simulink model "nonlin_feedback_simInput"  (R2023a)
settings: Solver=ode1  StartTime=0  StopTime=400  FixedStep=0.002  RelTol=1e-3
values from neighbouring files (symbols this model uses):
  B1 = [-kQ, -kQ, kQ, kQ ... (first row only)    [simulate_hover.m]
  B2 = [0, 0, 0 ... (first row only)    [simulate_hover.m]
  cycleGain = 0.2    [simulate_hover.m]    (also in temp.m = 1)
  I_xx = 0.0522    [simulate_hover.m]
  I_yy = 0.0522    [simulate_hover.m]
  I_zz = 0.1104    [simulate_hover.m]
  K = lqi(sys, Q, R)    [simulate_hover.m]
  k_T = 0.1188    [simulate_hover.m]
  kd = 0.5    [simulate_hover.m]
  kfr_p = 0.4*u2line/x5line    (= 0.285774113641)    [simulate_hover.m]
  kfr_r = 0.4*u1line/x4line    (= 0.285774113641)    [simulate_hover.m]
  kfr_y = 0.4*u3line/x6line    (= 0.0880063173321)    [simulate_hover.m]
  l_a = 0.1968    [simulate_hover.m]
  r = flexSize(no)    [phaseComp.m]    (also in simulate_hover.m = 0.5)
  sigma = 0    [simulate_hover.m]
  skew = 2    [simulate_hover.m]
  V_bias = 12    [setup_lab_hover.m]    (also in simulate_hover.m)
  velMax = 100*60*pi/180    (= 104.71975512)    [simulate_hover.m]
  VMAX_AMP = 24    [setup_lab_hover.m]    (also in simulate_hover.m)
  wcf = 2 * pi * 20    (= 125.663706144)    [setup_lab_hover.m]    (also in simulate_hover.m)
  zetaf = 0.6    [setup_lab_hover.m]    (also in simulate_hover.m)
undefined symbols (not defined in the file or in its folder): DG
libraries: simulink_extras x4, dspsrcs4 x1
settings Model: Creator=kille  LastModifiedBy=Jacob

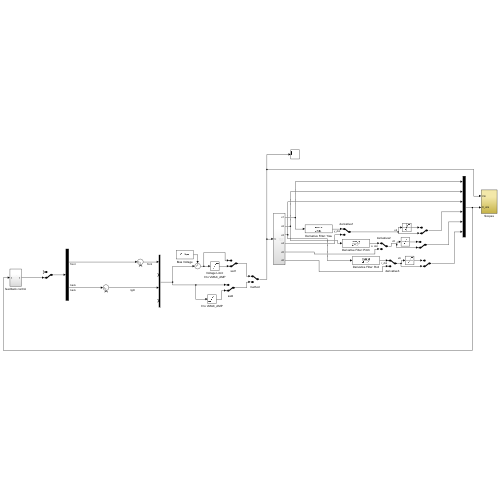
[thumbnail: Simulink's stored preview of the top-level diagram]
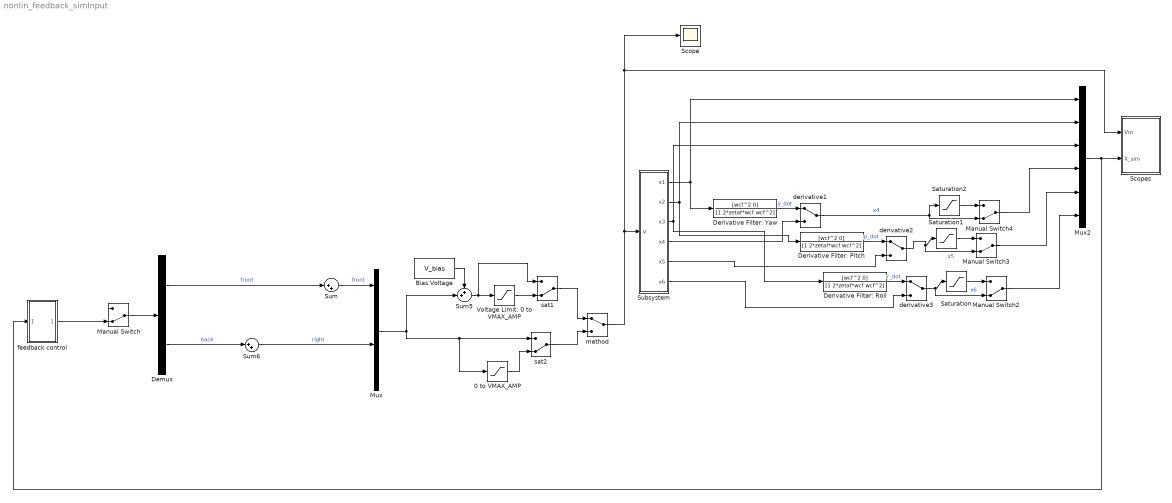
== system nonlin_feedback_simInput ==
  0 to VMAX_AMP : Saturate  UpperLimit=VMAX_AMP  LowerLimit=0
  Bias Voltage : Constant  Value=V_bias
  Demux : Demux  Outputs=2
  Derivative Filter: Pitch : TransferFcn  Numerator=[wcf^2 0]  Denominator=[1 2*zetaf*wcf wcf^2]
  Derivative Filter: Roll : TransferFcn  Numerator=[wcf^2 0]  Denominator=[1 2*zetaf*wcf wcf^2]
  Derivative Filter: Yaw : TransferFcn  Numerator=[wcf^2 0]  Denominator=[1 2*zetaf*wcf wcf^2]
  Manual Switch{,2..4} (4 alike) : ManualSwitch  CurrentSetting=0
  Mux : Mux
  Mux2 : Mux  Inputs=6
  Saturation : Saturate  UpperLimit=velMax  LowerLimit=-velMax
  Saturation1 : Saturate  UpperLimit=velMax  LowerLimit=-velMax
  Saturation2 : Saturate  UpperLimit=velMax  LowerLimit=-velMax
  Scope : Scope
  Scopes : Subsystem
  Subsystem : Subsystem
  Sum : Sum  Inputs=|++
  Sum5 : Sum  Inputs=++|
  Sum6 : Sum  Inputs=|++
  Voltage Limit: 0 to VMAX_AMP : Saturate  UpperLimit=VMAX_AMP  LowerLimit=0
  derivative1 : ManualSwitch
  derivative2 : ManualSwitch
  derivative3 : ManualSwitch
  feedback control : Subsystem
  method : ManualSwitch  Tag=swt
  sat1 : ManualSwitch  CurrentSetting=0
  sat2 : ManualSwitch  CurrentSetting=0
  wires:
  method/1 -> Scope/1, Scopes/1(Vm), Subsystem/1(V)
  sat2/1 -> method/2
  Mux/1 -> 0 to VMAX_AMP/1, sat2/1, Sum5/2
  Voltage Limit: 0 to VMAX_AMP/1 -> sat1/2
  Bias Voltage/1 -> Sum5/1
  Sum5/1 -> sat1/1, Voltage Limit: 0 to VMAX_AMP/1
  0 to VMAX_AMP/1 -> sat2/2
  sat1/1 -> method/1
  Sum/1 -> Mux/1  "front"
  Demux/1 -> Sum/1  "front"
  Sum6/1 -> Mux/3  "right"
  Derivative Filter: Yaw/1 -> derivative1/1  "y_dot"
  Derivative Filter: Pitch/1 -> derivative2/1  "p_dot"
  Derivative Filter: Roll/1 -> derivative3/1  "r_dot"
  Subsystem/1(x1) -> Mux2/1, Derivative Filter: Yaw/1
  Subsystem/4(x4) -> derivative1/2
  Subsystem/2(x2) -> Derivative Filter: Pitch/1, Mux2/2
  Subsystem/5(x5) -> derivative2/2
  Subsystem/6(x6) -> derivative3/2
  Subsystem/3(x3) -> Mux2/3, Derivative Filter: Roll/1
  Manual Switch4/1 -> Mux2/4
  Manual Switch2/1 -> Mux2/6
  Manual Switch3/1 -> Mux2/5
  Saturation/1 -> Manual Switch2/1
  derivative3/1 -> Manual Switch2/2, Saturation/1  "x6"
  Saturation1/1 -> Manual Switch3/1
  derivative2/1 -> Manual Switch3/2, Saturation1/1  "x5"
  Saturation2/1 -> Manual Switch4/1
  derivative1/1 -> Saturation2/1, Manual Switch4/2  "x4"
  Mux2/1 -> feedback control/1(In1), Scopes/2(X_sim)
  Demux/2 -> Sum6/1  "back"
  Manual Switch/1 -> Demux/1
  feedback control/1(Out1) -> Manual Switch/2

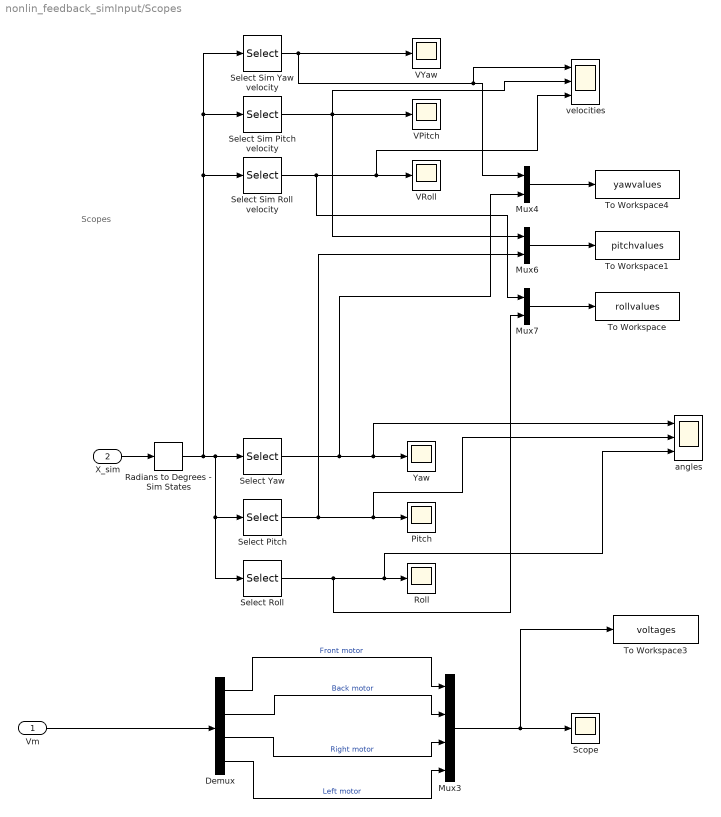
== system nonlin_feedback_simInput/Scopes ==
  note: Scopes
  Vm : Inport
  X_sim : Inport  Port=2
  Demux : Demux
  Mux3 : Mux
  Mux4 : Mux  Inputs=2
  Mux6 : Mux  Inputs=2
  Mux7 : Mux  Inputs=2
  Pitch : Scope
  Radians to Degrees - Sim States : simulink_extras/Transformations/Radians to Degrees
  Roll : Scope
  Scope : Scope
  Select Pitch : Selector  InputPortWidth=6  IndexOptions=Index vector (dialog)  Indices=2  OutputSizes=1
  Select Roll : Selector  InputPortWidth=6  IndexOptions=Index vector (dialog)  Indices=3  OutputSizes=1
  Select Sim Pitch velocity : Selector  InputPortWidth=6  IndexOptions=Index vector (dialog)  Indices=5  OutputSizes=1
  Select Sim Roll velocity : Selector  InputPortWidth=6  IndexOptions=Index vector (dialog)  Indices=6  OutputSizes=1
  Select Sim Yaw velocity : Selector  InputPortWidth=6  IndexOptions=Index vector (dialog)  Indices=4  OutputSizes=1
  Select Yaw : Selector  InputPortWidth=6  IndexOptions=Index vector (dialog)  Indices=1  OutputSizes=1
  To Workspace : ToWorkspace  VariableName=rollvalues  SampleTime=-1
  To Workspace1 : ToWorkspace  VariableName=pitchvalues  SampleTime=-1
  To Workspace3 : ToWorkspace  VariableName=voltages  SampleTime=-1
  To Workspace4 : ToWorkspace  VariableName=yawvalues  SampleTime=-1
  VPitch : Scope
  VRoll : Scope
  VYaw : Scope
  Yaw : Scope
  angles : Scope  NumInputPorts=3
  velocities : Scope  NumInputPorts=3
  wires:
  Select Roll/1 -> angles/3, Roll/1, Mux7/2
  Radians to Degrees - Sim States/1 -> Select Sim Roll velocity/1, Select Sim Pitch velocity/1, Select Sim Yaw velocity/1, Select Roll/1, Select Pitch/1, Select Yaw/1
  Select Pitch/1 -> angles/2, Pitch/1, Mux6/2
  X_sim/1 -> Radians to Degrees - Sim States/1
  Demux/1 -> Mux3/1  "Front motor"
  Demux/2 -> Mux3/2  "Back motor"
  Demux/3 -> Mux3/3  "Right motor"
  Demux/4 -> Mux3/4  "Left motor"
  Vm/1 -> Demux/1
  Select Sim Yaw velocity/1 -> VYaw/1, velocities/1, Mux4/1
  Select Sim Roll velocity/1 -> velocities/3, VRoll/1, Mux7/1
  Select Sim Pitch velocity/1 -> Mux6/1, velocities/2, VPitch/1
  Mux4/1 -> To Workspace4/1
  Mux6/1 -> To Workspace1/1
  Mux7/1 -> To Workspace/1
  Mux3/1 -> To Workspace3/1, Scope/1
  Select Yaw/1 -> angles/1, Yaw/1, Mux4/2

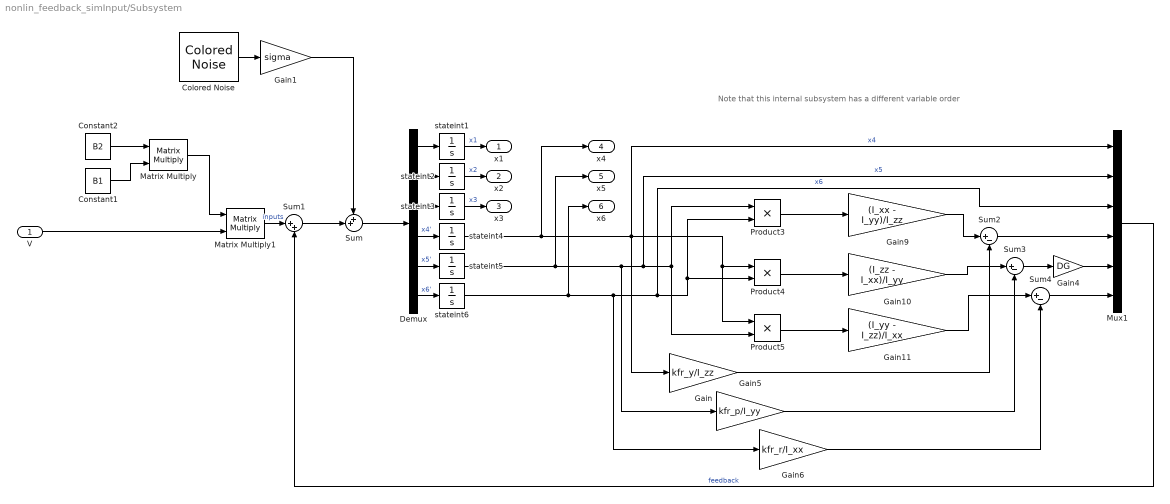
== system nonlin_feedback_simInput/Subsystem ==
  note: Note that this internal subsystem has a different variable order
  V : Inport
  Colored Noise : dspsrcs4/Colored Noise  Color=white  InverseFrequencyPower=1  BoundedOutput=off  NumChannels=6  OutputDataType=double  SamplesPerFrame=1  SampleTime=1  RandomStream=mt19937ar with seed  Seed=67  SimulateUsing=Interpreted execution
  Constant1 : Constant  Value=B1
  Constant2 : Constant  Value=B2
  Demux : Demux  Outputs=6
  Gain : Gain  Gain=kfr_y/I_zz
  Gain1 : Gain  Gain=sigma
  Gain10 : Gain  Gain=(I_zz - I_xx)/I_yy
  Gain11 : Gain  Gain=(I_yy - I_zz)/I_xx
  Gain4 : Gain  Gain=DG
  Gain5 : Gain  Gain=kfr_p/I_yy
  Gain6 : Gain  Gain=kfr_r/I_xx
  Gain9 : Gain  Gain=(I_xx - I_yy)/I_zz
  Matrix Multiply : Product  Multiplication=Matrix(*)
  Matrix Multiply1 : Product  Multiplication=Matrix(*)
  Mux1 : Mux  Inputs=6
  Product3 : Product
  Product4 : Product
  Product5 : Product
  Sum : Sum  Inputs=++|
  Sum1 : Sum  Inputs=|++
  Sum2 : Sum  Inputs=|+-
  Sum3 : Sum  Inputs=|+-
  Sum4 : Sum  Inputs=|+-
  stateint{1,4..6} (4 alike) : Integrator
  stateint2 : Integrator  InitialCondition=0.0005236
  stateint3 : Integrator  InitialCondition=0.0005236
  x1 : Outport
  x2 : Outport  Port=2
  x3 : Outport  Port=3
  x4 : Outport  Port=4
  x5 : Outport  Port=5
  x6 : Outport  Port=6
  wires:
  Mux1/1 -> Sum1/2  "feedback"
  stateint5/1 -> x5/1, Gain5/1, Mux1/2, Product5/2, Product3/1  "x5"
  Matrix Multiply1/1 -> Sum1/1  "inputs"
  stateint4/1 -> x4/1, Gain/1, Mux1/1, Product5/1, Product4/1  "x4"
  Matrix Multiply/1 -> Matrix Multiply1/1
  V/1 -> Matrix Multiply1/2
  Sum2/1 -> Mux1/4
  Gain6/1 -> Sum4/2
  Demux/1 -> stateint1/1
  stateint6/1 -> x6/1, Gain6/1, Mux1/3, Product4/2, Product3/2  "x6"
  Demux/6 -> stateint6/1  "x6'"
  Product5/1 -> Gain11/1
  Demux/5 -> stateint5/1  "x5'"
  Demux/2 -> stateint2/1
  Gain11/1 -> Sum4/1
  Constant1/1 -> Matrix Multiply/2
  Demux/3 -> stateint3/1
  Gain9/1 -> Sum2/1
  Gain10/1 -> Sum3/1
  Constant2/1 -> Matrix Multiply/1
  Demux/4 -> stateint4/1  "x4'"
  Product4/1 -> Gain10/1
  stateint1/1 -> x1/1  "x1"
  stateint2/1 -> x2/1  "x2"
  stateint3/1 -> x3/1  "x3"
  Colored Noise/1 -> Gain1/1
  Sum1/1 -> Sum/2
  Sum/1 -> Demux/1
  Gain1/1 -> Sum/1
  Product3/1 -> Gain9/1
  Gain/1 -> Sum2/2
  Gain5/1 -> Sum3/2
  Sum3/1 -> Gain4/1
  Sum4/1 -> Mux1/6
  Gain4/1 -> Mux1/5

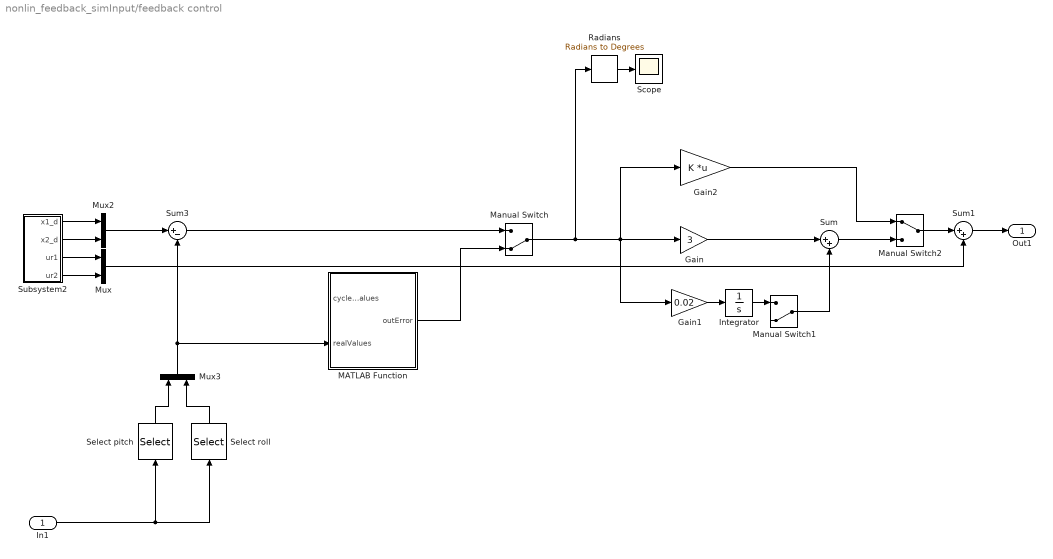
== system nonlin_feedback_simInput/feedback control ==
  In1 : Inport
  Gain : Gain  Gain=3
  Gain1 : Gain  Gain=0.02
  Gain2 : Gain  Gain=K  Multiplication=Matrix(K*u)
  Integrator : Integrator
  MATLAB Function : MATLAB Function  TreatAsAtomicUnit=on
  Manual Switch : ManualSwitch  CurrentSetting=0
  Manual Switch1 : ManualSwitch  CurrentSetting=0
  Manual Switch2 : ManualSwitch
  Mux : Mux  Inputs=2
  Mux2 : Mux  Inputs=2
  Mux3 : Mux  Inputs=2
  Radians : simulink_extras/Transformations/Radians to Degrees
  Scope : Scope
  Select pitch : Selector  InputPortWidth=6  IndexOptions=Index vector (dialog)  Indices=2  OutputSizes=1
  Select roll : Selector  InputPortWidth=6  IndexOptions=Index vector (dialog)  Indices=3  OutputSizes=1
  Subsystem2 : Subsystem
  Sum : Sum  Inputs=|++
  Sum1 : Sum  Inputs=|++
  Sum3 : Sum  Inputs=|+-
  Out1 : Outport
  wires:
  Mux3/1 -> MATLAB Function/2(realValues), Sum3/2
  In1/1 -> Select roll/1, Select pitch/1
  Mux2/1 -> Sum3/1
  Select pitch/1 -> Mux3/1
  Subsystem2/1(x1_d) -> Mux2/1
  Subsystem2/2(x2_d) -> Mux2/2
  Select roll/1 -> Mux3/2
  Gain/1 -> Sum/1
  Gain1/1 -> Integrator/1
  Integrator/1 -> Manual Switch1/1
  Manual Switch1/1 -> Sum/2
  Sum3/1 -> Manual Switch/1
  MATLAB Function/1(outError) -> Manual Switch/2
  Sum/1 -> Manual Switch2/2
  Gain2/1 -> Manual Switch2/1
  Manual Switch/1 -> Radians/1, Gain2/1, Gain1/1, Gain/1
  Radians/1 -> Scope/1
  Subsystem2/3(ur1) -> Mux/1
  Subsystem2/4(ur2) -> Mux/2
  Mux/1 -> Sum1/2
  Manual Switch2/1 -> Sum1/1
  Sum1/1 -> Out1/1

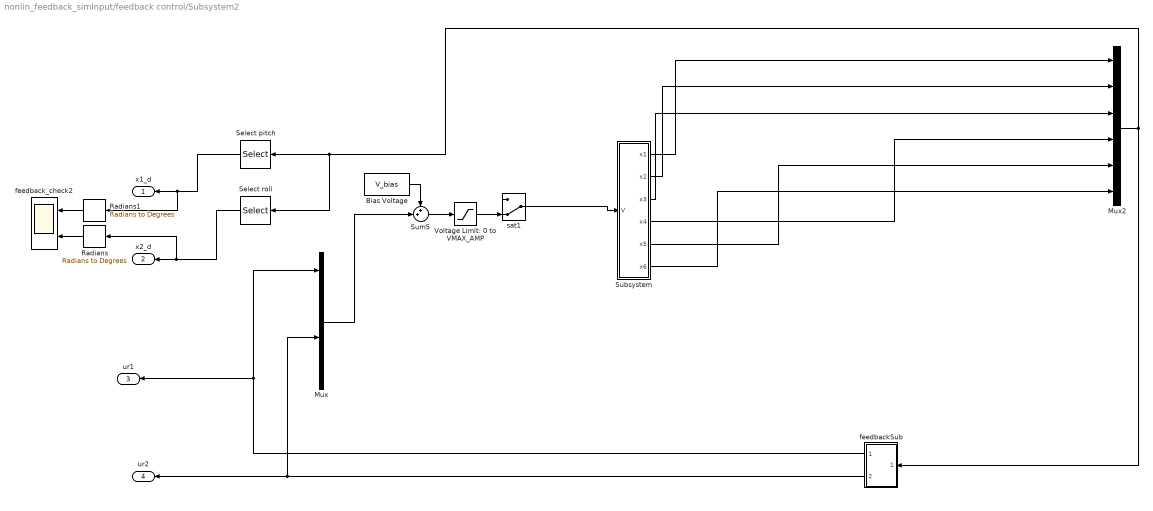
== system nonlin_feedback_simInput/feedback control/Subsystem2 ==
  Bias Voltage : Constant  Value=V_bias
  Mux : Mux
  Mux2 : Mux  Inputs=6
  Radians : simulink_extras/Transformations/Radians to Degrees
  Radians1 : simulink_extras/Transformations/Radians to Degrees
  Select pitch : Selector  InputPortWidth=6  IndexOptions=Index vector (dialog)  Indices=2  OutputSizes=1
  Select roll : Selector  InputPortWidth=6  IndexOptions=Index vector (dialog)  Indices=3  OutputSizes=1
  Subsystem : Subsystem
  Sum5 : Sum  Inputs=++|
  Voltage Limit: 0 to VMAX_AMP : Saturate  UpperLimit=VMAX_AMP  LowerLimit=0
  feedbackSub : Subsystem
  feedback_check2 : Scope  NumInputPorts=2
  sat1 : ManualSwitch  CurrentSetting=0
  x1_d : Outport
  x2_d : Outport  Port=2
  ur1 : Outport  Port=3
  ur2 : Outport  Port=4
  wires:
  Radians1/1 -> feedback_check2/1
  Radians/1 -> feedback_check2/2
  Bias Voltage/1 -> Sum5/1
  Mux2/1 -> feedbackSub/1(Input), Select roll/1, Select pitch/1
  Subsystem/1(x1) -> Mux2/1
  Sum5/1 -> Voltage Limit: 0 to VMAX_AMP/1
  Subsystem/2(x2) -> Mux2/2
  Subsystem/3(x3) -> Mux2/3
  sat1/1 -> Subsystem/1(V)
  Voltage Limit: 0 to VMAX_AMP/1 -> sat1/2
  Mux/1 -> Sum5/2
  feedbackSub/1(ur1) -> ur1/1, Mux/1
  feedbackSub/2(ur2) -> ur2/1, Mux/3
  Select roll/1 -> Radians/1, x2_d/1
  Select pitch/1 -> Radians1/1, x1_d/1
  Subsystem/4(x4) -> Mux2/4
  Subsystem/5(x5) -> Mux2/5
  Subsystem/6(x6) -> Mux2/6

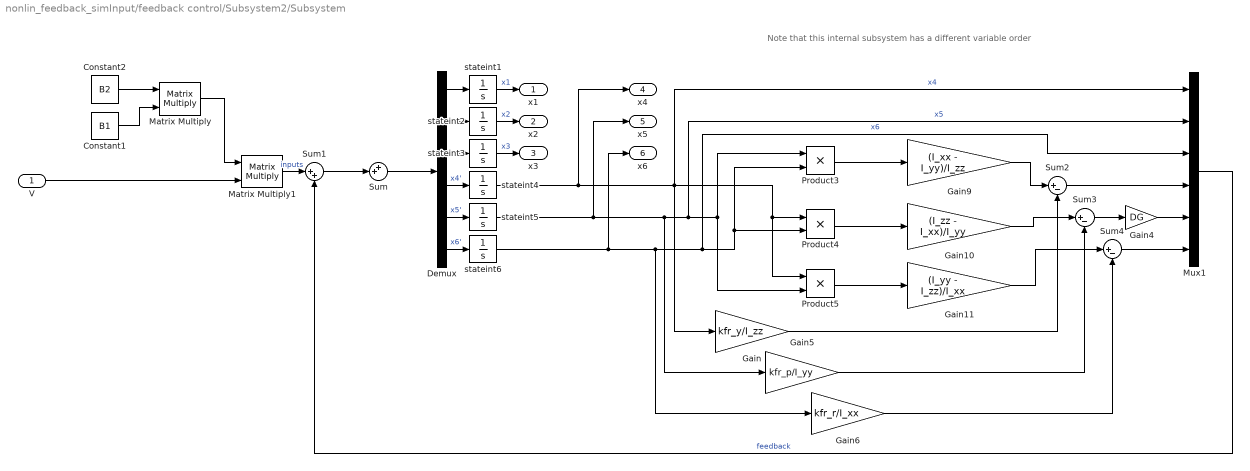
== system nonlin_feedback_simInput/feedback control/Subsystem2/Subsystem ==
  note: Note that this internal subsystem has a different variable order
  V : Inport
  Constant1 : Constant  Value=B1
  Constant2 : Constant  Value=B2
  Demux : Demux  Outputs=6
  Gain : Gain  Gain=kfr_y/I_zz
  Gain10 : Gain  Gain=(I_zz - I_xx)/I_yy
  Gain11 : Gain  Gain=(I_yy - I_zz)/I_xx
  Gain4 : Gain  Gain=DG
  Gain5 : Gain  Gain=kfr_p/I_yy
  Gain6 : Gain  Gain=kfr_r/I_xx
  Gain9 : Gain  Gain=(I_xx - I_yy)/I_zz
  Matrix Multiply : Product  Multiplication=Matrix(*)
  Matrix Multiply1 : Product  Multiplication=Matrix(*)
  Mux1 : Mux  Inputs=6
  Product3 : Product
  Product4 : Product
  Product5 : Product
  Sum : Sum  Inputs=++|
  Sum1 : Sum  Inputs=|++
  Sum2 : Sum  Inputs=|+-
  Sum3 : Sum  Inputs=|+-
  Sum4 : Sum  Inputs=|+-
  stateint{1,4..6} (4 alike) : Integrator
  stateint2 : Integrator  InitialCondition=0.0005236
  stateint3 : Integrator  InitialCondition=0.0005236
  x1 : Outport
  x2 : Outport  Port=2
  x3 : Outport  Port=3
  x4 : Outport  Port=4
  x5 : Outport  Port=5
  x6 : Outport  Port=6
  wires:
  Mux1/1 -> Sum1/2  "feedback"
  stateint5/1 -> x5/1, Gain5/1, Mux1/2, Product5/2, Product3/1  "x5"
  Matrix Multiply1/1 -> Sum1/1  "inputs"
  stateint4/1 -> x4/1, Gain/1, Mux1/1, Product5/1, Product4/1  "x4"
  Matrix Multiply/1 -> Matrix Multiply1/1
  V/1 -> Matrix Multiply1/2
  Sum2/1 -> Mux1/4
  Gain6/1 -> Sum4/2
  Demux/1 -> stateint1/1
  stateint6/1 -> x6/1, Gain6/1, Mux1/3, Product4/2, Product3/2  "x6"
  Demux/6 -> stateint6/1  "x6'"
  Product5/1 -> Gain11/1
  Demux/5 -> stateint5/1  "x5'"
  Demux/2 -> stateint2/1
  Gain11/1 -> Sum4/1
  Constant1/1 -> Matrix Multiply/2
  Demux/3 -> stateint3/1
  Gain9/1 -> Sum2/1
  Gain10/1 -> Sum3/1
  Constant2/1 -> Matrix Multiply/1
  Demux/4 -> stateint4/1  "x4'"
  Product4/1 -> Gain10/1
  stateint1/1 -> x1/1  "x1"
  stateint2/1 -> x2/1  "x2"
  stateint3/1 -> x3/1  "x3"
  Sum1/1 -> Sum/2
  Sum/1 -> Demux/1
  Product3/1 -> Gain9/1
  Gain/1 -> Sum2/2
  Gain5/1 -> Sum3/2
  Sum3/1 -> Gain4/1
  Sum4/1 -> Mux1/6
  Gain4/1 -> Mux1/5

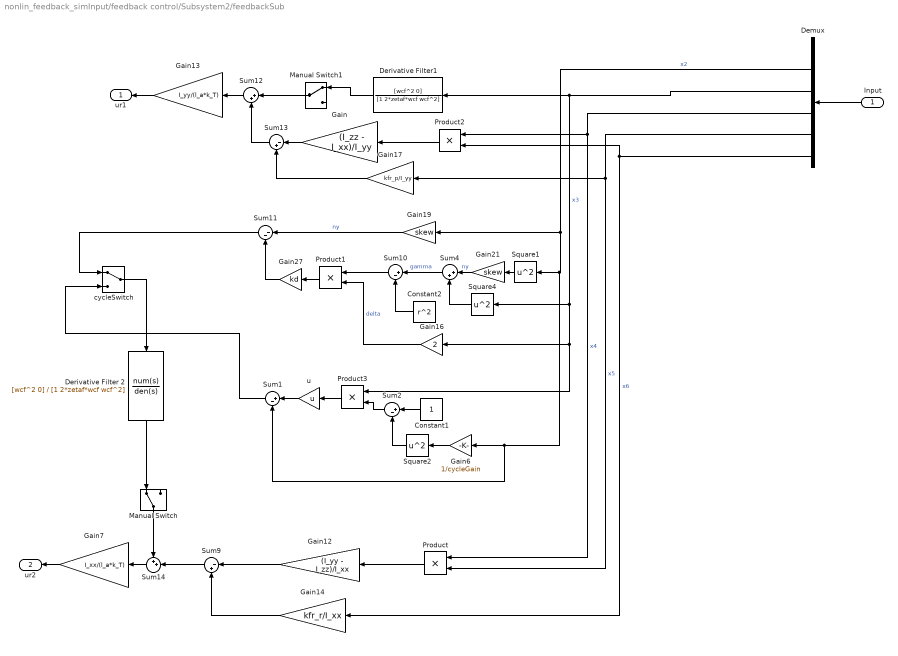
== system nonlin_feedback_simInput/feedback control/Subsystem2/feedbackSub ==
  Input : Inport
  Constant1 : Constant
  Constant2 : Constant  Value=r^2
  Demux : Demux  Outputs=6
  Derivative Filter 2 : TransferFcn  Numerator=[wcf^2 0]  Denominator=[1 2*zetaf*wcf wcf^2]
  Derivative Filter1 : TransferFcn  Numerator=[wcf^2 0]  Denominator=[1 2*zetaf*wcf wcf^2]
  Gain : Gain  Gain=(I_zz - I_xx)/I_yy
  Gain12 : Gain  Gain=(I_yy - I_zz)/I_xx
  Gain13 : Gain  Gain=I_yy/(l_a*k_T)
  Gain14 : Gain  Gain=kfr_r/I_xx
  Gain16 : Gain  Gain=2
  Gain17 : Gain  Gain=kfr_p/I_yy
  Gain19 : Gain  Gain=skew
  Gain21 : Gain  Gain=skew
  Gain27 : Gain  Gain=kd
  Gain6 : Gain  Gain=1/cycleGain
  Gain7 : Gain  Gain=I_xx/(l_a*k_T)
  Manual Switch : ManualSwitch
  Manual Switch1 : ManualSwitch
  Product{,1..3} (4 alike) : Product
  Square1 : Math  Operator=square
  Square2 : Math  Operator=square
  Square4 : Math  Operator=square
  Sum1 : Sum  Inputs=|+-
  Sum10 : Sum  Inputs=|+-
  Sum11 : Sum  Inputs=|--
  Sum12 : Sum  Inputs=|++
  Sum13 : Sum  Inputs=|-+
  Sum14 : Sum  Inputs=++|
  Sum2 : Sum  Inputs=|+-
  Sum4 : Sum  Inputs=|++
  Sum9 : Sum  Inputs=|-+
  cycleSwitch : ManualSwitch
  u : Gain  Gain=u
  ur1 : Outport
  ur2 : Outport  Port=2
  wires:
  Derivative Filter1/1 -> Manual Switch1/1
  Gain17/1 -> Sum13/2
  Sum13/1 -> Sum12/2
  Demux/4 -> Product/1, Product2/1  "x4"
  Gain21/1 -> Sum4/1  "ny"
  Product2/1 -> Gain/1
  Sum12/1 -> Gain13/1
  Demux/5 -> Product/2, Gain17/1  "x5"
  Sum14/1 -> Gain7/1
  Gain27/1 -> Sum11/2
  Product/1 -> Gain12/1
  Constant2/1 -> Sum10/2
  Sum10/1 -> Product1/1
  Demux/6 -> Gain14/1, Product2/2  "x6"
  Manual Switch/1 -> Sum14/1
  Manual Switch1/1 -> Sum12/1
  Sum4/1 -> Sum10/1  "gamma"
  Sum9/1 -> Sum14/2
  Square4/1 -> Sum4/2
  Gain12/1 -> Sum9/1
  Square1/1 -> Gain21/1
  Product1/1 -> Gain27/1
  Gain/1 -> Sum13/1
  Gain14/1 -> Sum9/2
  Gain13/1 -> ur1/1
  Gain19/1 -> Sum11/1  "ny"
  Gain16/1 -> Product1/2  "delta"
  Derivative Filter 2/1 -> Manual Switch/1
  Gain7/1 -> ur2/1
  Input/1 -> Demux/1
  Square2/1 -> Sum2/2
  Demux/2 -> Gain19/1, Gain6/1, Sum1/2, Square1/1  "x2"
  Constant1/1 -> Sum2/1
  Sum2/1 -> Product3/2
  Product3/1 -> u/1
  Gain6/1 -> Square2/1
  Demux/3 -> Derivative Filter1/1, Square4/1, Product3/1, Gain16/1  "x3"
  u/1 -> Sum1/1
  Sum11/1 -> cycleSwitch/1
  cycleSwitch/1 -> Derivative Filter 2/1
  Sum1/1 -> cycleSwitch/2

== matlab function nonlin_feedback_simInput/feedback control/MATLAB Function ==
  data: cycleValues input; realValues input; outError output
function outError = approxLimitSimu(cycleValues, realValues)
    outError = transpose([0, 0]);
    %temp = load('paperCycle.mat');
    %cycleValues = temp.paperCycle;
    %for n = 1:2
    %    cycleN = cycleValues(:, n);
    %    realValueN = realValues(n);
    %    [closestValueError,idx]=min(abs(cycleN-realValueN));
    %    outError(n) = closestValueError;
    %end
    %disp(length(cycleValues))
    coder.extrinsic('approxLimit');
    outError = transpose(approxLimit(realValues));
